simulink model "Modele_LQR_6DOF"  (R2025b)
settings: Solver=VariableStepAuto  StartTime=0.0  StopTime=300  FixedStep=0.033333  RelTol=1e-3
values from neighbouring files (symbols this model uses):
  B = -234.459    [AUV_Params.sldd]    (also in block_compute_K.m = [ [                                          0,             )
  Fx1 = -14.142    [AUV_Params.sldd]
  Fx2 = -14.142    [AUV_Params.sldd]
  Fx3 = 0.0    [AUV_Params.sldd]
  Fx4 = 0.0    [AUV_Params.sldd]
  Fx5 = 0.0    [AUV_Params.sldd]
  Fx6 = 0.0    [AUV_Params.sldd]
  Fx7 = 14.142    [AUV_Params.sldd]
  Fx8 = 14.142    [AUV_Params.sldd]
  Fy1 = 14.142    [AUV_Params.sldd]
  Fy2 = -14.142    [AUV_Params.sldd]
  Fy3 = 0.0    [AUV_Params.sldd]
  Fy4 = 0.0    [AUV_Params.sldd]
  Fy5 = 0.0    [AUV_Params.sldd]
  Fy6 = 0.0    [AUV_Params.sldd]
  Fy7 = 14.142    [AUV_Params.sldd]
  Fy8 = -14.142    [AUV_Params.sldd]
  Fz1 = 0.0    [AUV_Params.sldd]
  Fz2 = 0.0    [AUV_Params.sldd]
  Fz3 = -20.0    [AUV_Params.sldd]
  Fz4 = -20.0    [AUV_Params.sldd]
  Fz5 = -20.0    [AUV_Params.sldd]
  Fz6 = -20.0    [AUV_Params.sldd]
  Fz7 = 0.0    [AUV_Params.sldd]
  Fz8 = 0.0    [AUV_Params.sldd]
  I_x = 0.578    [AUV_Params.sldd]
  I_y = 0.645    [AUV_Params.sldd]
  I_z = 0.9366    [AUV_Params.sldd]
  lx1 = 0.0194    [AUV_Params.sldd]
  lx2 = 0.0194    [AUV_Params.sldd]
  lx3 = -0.0317    [AUV_Params.sldd]
  lx4 = -0.0317    [AUV_Params.sldd]
  lx5 = 0.0317    [AUV_Params.sldd]
  lx6 = 0.0317    [AUV_Params.sldd]
  lx7 = -0.0194    [AUV_Params.sldd]
  lx8 = -0.0194    [AUV_Params.sldd]
  ly1 = 0.0381    [AUV_Params.sldd]
  ly2 = -0.0381    [AUV_Params.sldd]
  ly3 = 0.0049    [AUV_Params.sldd]
  ly4 = -0.0049    [AUV_Params.sldd]
  ly5 = 0.0049    [AUV_Params.sldd]
  ly6 = -0.0049    [AUV_Params.sldd]
  ly7 = 0.0381    [AUV_Params.sldd]
  ly8 = -0.0381    [AUV_Params.sldd]
  lz1 = 0.0575    [AUV_Params.sldd]
  lz2 = 0.0575    [AUV_Params.sldd]
  lz3 = 0.0366    [AUV_Params.sldd]
  lz4 = 0.0366    [AUV_Params.sldd]
  lz5 = 0.0366    [AUV_Params.sldd]
  lz6 = 0.0366    [AUV_Params.sldd]
  lz7 = 0.0575    [AUV_Params.sldd]
  lz8 = 0.0575    [AUV_Params.sldd]
  m = 23.9    [AUV_Params.sldd]
  W = 234.459    [AUV_Params.sldd]
  x_rb = 0.0    [AUV_Params.sldd]
  x_rg = 0.0    [AUV_Params.sldd]
  y_rb = 0.0    [AUV_Params.sldd]
  y_rg = 0.0    [AUV_Params.sldd]
  z_rb = 0.0    [AUV_Params.sldd]
  z_rg = 0.0    [AUV_Params.sldd]
undefined symbols (not defined in the file or in its folder): A_num, Q_envoyer, sigbuilder_block, SIZE_TRAJ, T_TRAJ, TRAJECTOIRE, YAW_MODE
libraries: simulink x12, sharedtransform x1, dspinverses x1, SignalEditorBlockLib x1
(part 3 of 4)

== matlab function Modele_LQR_6DOF/Controller/MATLAB Function ==
  settings: updateMethod=DISCRETE
  data: R output; Q output; A output; B output; state input; Q_files input; A_lineraire input

function [R,Q,A,B]= ABmatrix(state, Q_files, A_lineraire)
tic
    
    roll_ = state(4);
    pitch_ = state(5);
    yaw_ = state(6);
    u = state(7); %
    v = state(8); %
    w = state(9); %
    p = state(10);
    q = state(11);
    r = state(12);
    thrust = 10;
    importance = 0;

    % Q = Q_files;
    Q = diag([Q_files(1,1) Q_files(2,2) Q_files(3,3) Q_files(4,4) Q_files(5,5) Q_files(6,6) Q_files(7,7) Q_files(8,8) Q_files(9,9) Q_files(10,10) Q_files(11,11) Q_files(12,12)]);
    % Q = diag([80, 80, 80, 40, 40, 40, 20, 20, 20, 20, 20, 20]); % test répétition
    % Q = diag([4, 4, 4, 2, 2, 2, 1, 1, 1, 1, 1, 1]); % test ancien
    % R = diag([thrust, thrust, thrust-importance, thrust-importance, thrust-importance, thrust-importance, thrust, thrust]); 
    R = thrust*eye(8);

    radius = 0.26;
    
 % A = A_lineraire;

 A = [[0, 0, 0,   v*(sin(roll_)*sin(yaw_) + cos(roll_)*cos(yaw_)*sin(pitch_)) + w*(cos(roll_)*sin(yaw_) - cos(yaw_)*sin(pitch_)*sin(roll_)), w*cos(pitch_)*cos(roll_)*cos(yaw_) - u*cos(yaw_)*sin(pitch_) + v*cos(pitch_)*cos(yaw_)*sin(roll_), w*(cos(yaw_)*sin(roll_) - cos(roll_)*sin(pitch_)*sin(yaw_)) - v*(cos(roll_)*cos(yaw_) + sin(pitch_)*sin(roll_)*sin(yaw_)) - u*cos(pitch_)*sin(yaw_), cos(pitch_)*cos(yaw_), cos(yaw_)*sin(pitch_)*sin(roll_) - cos(roll_)*sin(yaw_), sin(roll_)*sin(yaw_) + cos(roll_)*cos(yaw_)*sin(pitch_),             0,                      0,                      0]
[0, 0, 0, - v*(cos(yaw_)*sin(roll_) - cos(roll_)*sin(pitch_)*sin(yaw_)) - w*(cos(roll_)*cos(yaw_) + sin(pitch_)*sin(roll_)*sin(yaw_)), w*cos(pitch_)*cos(roll_)*sin(yaw_) - u*sin(pitch_)*sin(yaw_) + v*cos(pitch_)*sin(roll_)*sin(yaw_), w*(sin(roll_)*sin(yaw_) + cos(roll_)*cos(yaw_)*sin(pitch_)) - v*(cos(roll_)*sin(yaw_) - cos(yaw_)*sin(pitch_)*sin(roll_)) + u*cos(pitch_)*cos(yaw_), cos(pitch_)*sin(yaw_), cos(roll_)*cos(yaw_) + sin(pitch_)*sin(roll_)*sin(yaw_), cos(roll_)*sin(pitch_)*sin(yaw_) - cos(yaw_)*sin(roll_),             0,                      0,                      0]
[0, 0, 0,                                                                         v*cos(pitch_)*cos(roll_) - w*cos(pitch_)*sin(roll_),                             - u*cos(pitch_) - w*cos(roll_)*sin(pitch_) - v*sin(pitch_)*sin(roll_),                                                                                                                                                   0,          -sin(pitch_),                                  cos(pitch_)*sin(roll_),                                  cos(pitch_)*cos(roll_),             0,                      0,                      0]
[0, 0, 0,                                                                         q*cos(roll_)*tan(pitch_) - r*tan(pitch_)*sin(roll_),                               r*cos(roll_)*(tan(pitch_)^2 + 1) + q*sin(roll_)*(tan(pitch_)^2 + 1),                                                                                                                                                   0,                     0,                                                       0,                                                       0,             1, tan(pitch_)*sin(roll_), cos(roll_)*tan(pitch_)]
[0, 0, 0,                                                                                               - r*cos(roll_) - q*sin(roll_),                                                                                                 0,                                                                                                                                                   0,                     0,                                                       0,                                                       0,             0,             cos(roll_),            -sin(roll_)]
[0, 0, 0,                                                                     (q*cos(roll_))/cos(pitch_) - (r*sin(roll_))/cos(pitch_),               (r*cos(roll_)*sin(pitch_))/cos(pitch_)^2 + (q*sin(pitch_)*sin(roll_))/cos(pitch_)^2,                                                                                                                                                   0,                     0,                                                       0,                                                       0,             0, sin(roll_)/cos(pitch_), cos(roll_)/cos(pitch_)]
[0, 0, 0,                                                                                                                           0,                                            (10*cos(pitch_)*(13080*pi*radius^3 - 234459/1000))/139,                                                                                                                                                   0,            -2221/1390,                                                       r,                                                      -q,             0,                     -w,                      v]
[0, 0, 0,                                                          -(10*cos(pitch_)*cos(roll_)*(13080*pi*radius^3 - 234459/1000))/139,                                 (10*sin(pitch_)*sin(roll_)*(13080*pi*radius^3 - 234459/1000))/139,                                                                                                                                                   0,                    -r,                                               -1394/695,                                                       p,             w,                      0,                     -u]
[0, 0, 0,                                                           (10*cos(pitch_)*sin(roll_)*(13080*pi*radius^3 - 234459/1000))/139,                                 (10*cos(roll_)*sin(pitch_)*(13080*pi*radius^3 - 234459/1000))/139,                                                                                                                                                   0,                     q,                                                      -p,                                               -2107/695,            -v,                      u,                      0]
[0, 0, 0,                                                                                                                           0,                                                                                                 0,                                                                                                                                                   0,                     0,                                                       0,                                                       0, -193590/40171,           -(146*r)/289,           -(146*q)/289]
[0, 0, 0,                                                                                                                           0,                                                                                                 0,                                                                                                                                                   0,                     0,                                                       0,                                                       0,   (359*r)/645,            -25812/5977,            (359*p)/645]
[0, 0, 0,                                                                                                                           0,                                                                                                 0,                                                                                                                                                   0,                     0,                                                       0,                                                       0,   -(67*q)/937,            -(67*p)/937,         -387180/130243]];

% original
%     A = [[ 0, 0, 0,   v*(sin(roll_)*sin(yaw_) + cos(roll_)*cos(yaw_)*sin(pitch_)) + w*(cos(roll_)*sin(yaw_) - cos(yaw_)*sin(pitch_)*sin(roll_)), w*cos(pitch_)*cos(roll_)*cos(yaw_) - u*cos(yaw_)*sin(pitch_) + v*cos(pitch_)*cos(yaw_)*sin(roll_), w*(cos(yaw_)*sin(roll_) - cos(roll_)*sin(pitch_)*sin(yaw_)) - v*(cos(roll_)*cos(yaw_) + sin(pitch_)*sin(roll_)*sin(yaw_)) - u*cos(pitch_)*sin(yaw_), cos(pitch_)*cos(yaw_), cos(yaw_)*sin(pitch_)*sin(roll_) - cos(roll_)*sin(yaw_), sin(roll_)*sin(yaw_) + cos(roll_)*cos(yaw_)*sin(pitch_),          0,                      0,                      0]
% [ 0, 0, 0, - v*(cos(yaw_)*sin(roll_) - cos(roll_)*sin(pitch_)*sin(yaw_)) - w*(cos(roll_)*cos(yaw_) + sin(pitch_)*sin(roll_)*sin(yaw_)), w*cos(pitch_)*cos(roll_)*sin(yaw_) - u*sin(pitch_)*sin(yaw_) + v*cos(pitch_)*sin(roll_)*sin(yaw_), w*(sin(roll_)*sin(yaw_) + cos(roll_)*cos(yaw_)*sin(pitch_)) - v*(cos(roll_)*sin(yaw_) - cos(yaw_)*sin(pitch_)*sin(roll_)) + u*cos(pitch_)*cos(yaw_), cos(pitch_)*sin(yaw_), cos(roll_)*cos(yaw_) + sin(pitch_)*sin(roll_)*sin(yaw_), cos(roll_)*sin(pitch_)*sin(yaw_) - cos(yaw_)*sin(roll_),          0,                      0,                      0]
% [ 0, 0, 0,                                                                         v*cos(pitch_)*cos(roll_) - w*cos(pitch_)*sin(roll_),                             - u*cos(pitch_) - w*cos(roll_)*sin(pitch_) - v*sin(pitch_)*sin(roll_),                                                                                                                                                   0,          -sin(pitch_),                                  cos(pitch_)*sin(roll_),                                  cos(pitch_)*cos(roll_),          0,                      0,                      0]
% [ 0, 0, 0,                                                                         q*cos(roll_)*tan(pitch_) - r*tan(pitch_)*sin(roll_),                               r*cos(roll_)*(tan(pitch_)^2 + 1) + q*sin(roll_)*(tan(pitch_)^2 + 1),                                                                                                                                                   0,                     0,                                                       0,                                                       0,          1, tan(pitch_)*sin(roll_), cos(roll_)*tan(pitch_)]
% [ 0, 0, 0,                                                                                               - r*cos(roll_) - q*sin(roll_),                                                                                                 0,                                                                                                                                                   0,                     0,                                                       0,                                                       0,          0,             cos(roll_),            -sin(roll_)]
% [ 0, 0, 0,                                                                     (q*cos(roll_))/cos(pitch_) - (r*sin(roll_))/cos(pitch_),               (r*cos(roll_)*sin(pitch_))/cos(pitch_)^2 + (q*sin(pitch_)*sin(roll_))/cos(pitch_)^2,                                                                                                                                                   0,                     0,                                                       0,                                                       0,          0, sin(roll_)/cos(pitch_), cos(roll_)/cos(pitch_)]
% [ 0, 0, 0,                                                                                                                           0,                                                    (7873445366256113*cos(pitch_))/395824185999360,                                                                                                                                                   0,             2221/2250,                                               (17*r)/25,                                          -(1343*q)/2250,          0,         -(1343*w)/2250,              (17*v)/25]
% [ 0, 0, 0,                                                                   -(2315719225369445*cos(pitch_)*cos(roll_))/79164837199872,                                          (2315719225369445*sin(pitch_)*sin(roll_))/79164837199872,                                                                                                                                                   0,            -(25*r)/17,                                                   82/45,                                               (79*p)/90,  (79*w)/90,                      0,             -(25*u)/17]
% [ 0, 0, 0,                                                                      (146564507934775*cos(pitch_)*sin(roll_))/4398046511104,                                            (146564507934775*cos(roll_)*sin(pitch_))/4398046511104,                                                                                                                                                   0,         (2250*q)/1343,                                              -(90*p)/79,                                               4214/1343, -(90*v)/79,          (2250*u)/1343,                      0]
% [ 0, 0, 0,                                                                                                                           0,                                                                                                 0,                                                                                                                                                   0,                     0,                                               (187*w)/4,                                               (187*v)/4,       81/2,                      0,                      0]
% [ 0, 0, 0,                                                                                                                           0,                                                                                                 0,                                                                                                                                                   0,            -(907*w)/4,                                                       0,                                              -(907*u)/4,          0,                   81/2,                      0]
% [ 0, 0, 0,                                                                                                                           0,                                                                                                 0,                                                                                                                                                   0,                 180*v,                                                   180*u,                                                       0,          0,                      0,                   81/2]];


    B = [[                                          0,                                            0,              0,              0,             0,             0,                                            0,                                           0]
[                                          0,                                            0,              0,              0,             0,             0,                                            0,                                           0]
[                                          0,                                            0,              0,              0,             0,             0,                                            0,                                           0]
[                                          0,                                            0,              0,              0,             0,             0,                                            0,                                           0]
[                                          0,                                            0,              0,              0,             0,             0,                                            0,                                           0]
[                                          0,                                            0,              0,              0,             0,             0,                                            0,                                           0]
[                                  -707/6950,                                    -707/6950,              0,              0,             0,             0,                                     707/6950,                                    707/6950]
[                                   707/6950,                                    -707/6950,              0,              0,             0,             0,                                     707/6950,                                   -707/6950]
[                                          0,                                            0,        -20/139,        -20/139,       -20/139,       -20/139,                                            0,                                           0]
[                                          0,                                            0,  -130255/80342,   130255/80342, -130255/80342,  130255/80342,                                            0,                                           0]
[                                          0,                                            0, -256447/448275, -256447/448275, 256447/448275, 256447/448275,                                            0,                                           0]
[194698457386957391875/146640581566903877632, -194698457386957391875/146640581566903877632,              0,              0,             0,             0, -194698457386957391875/146640581566903877632, 194698457386957391875/146640581566903877632]];

% matrice original
%     B = [[                                   0,                                    0,         0,         0,         0,         0,                                    0,                                   0]
% [                                   0,                                    0,         0,         0,         0,         0,                                    0,                                   0]
% [                                   0,                                    0,         0,         0,         0,         0,                                    0,                                   0]
% [                                   0,                                    0,         0,         0,         0,         0,                                    0,                                   0]
% [                                   0,                                    0,         0,         0,         0,         0,                                    0,                                   0]
% [                                   0,                                    0,         0,         0,         0,         0,                                    0,                                   0]
% [                          -707/11250,                           -707/11250,         0,         0,         0,         0,                            707/11250,                           707/11250]
% [                            707/7650,                            -707/7650,         0,         0,         0,         0,                             707/7650,                           -707/7650]
% [                                   0,                                    0, -200/1343, -200/1343, -200/1343, -200/1343,                                    0,                                   0]
% [                                   0,                                    0,    -109/8,     109/8,    -109/8,     109/8,                                    0,                                   0]
% [                                   0,                                    0, -1073/200, -1073/200,  1073/200,  1073/200,                                    0,                                   0]
% [ 162927579403311625/9007199254740992, -162927579403311625/9007199254740992,         0,         0,         0,         0, -162927579403311625/9007199254740992, 162927579403311625/9007199254740992]];

toc
end

== matlab function Modele_LQR_6DOF/Thrustherforces in newtons/MATLAB Function1 ==
  data: u input; y output
function y = Normalize(u)
y = (u-1500)*150/400;

== matlab function Modele_LQR_6DOF/ROV model/ROV model/Kinematics ==
  data: u_b input; u_n output; v_b input; w_b input; p_b input; q_b input; r_b input; phi input; theta input; psi input; v_n output; w_n output; p_n output; q_n output; r_n output
function [u_n,v_n,w_n,p_n,q_n,r_n] = Kinematics(u_b,v_b,w_b,p_b,q_b,r_b,phi,theta,psi)
% LIVRE HMCH PAGE 27
cphi = cos(phi);
sphi = sin(phi);
cth  = cos(theta);
sth  = sin(theta);
cpsi = cos(psi);
spsi = sin(psi);
tanth = tan(theta);
if cth==0
    error('T is singular for theta = +-90 degrees');
end
 
u_n = u_b*cpsi*cth + v_b*(cpsi*sphi*sth - cphi*spsi) + w_b*(sphi*spsi + cphi*cpsi*sth) ;
v_n = u_b*cth*spsi + v_b*(cphi*cpsi + sphi*spsi*sth) + w_b*(cphi*spsi*sth - cpsi*sphi);
w_n = -u_b*sth+ v_b*cth*sphi + w_b*cphi*cth;
p_n = p_b + q_b*sphi*(tanth) + r_b*cphi*(tanth);
q_n = q_b*cphi - r_b*sphi;
r_n = q_b*(sphi/cth) + r_b*(cphi/cth);

% u_n =  w_b*(sphi*spsi + cphi*cpsi*sth) - v_b*(cphi*spsi - cpsi*sphi*sth) + u_b*cpsi*cth;
% v_n =  v_b*(cphi*cpsi + sphi*spsi*sth) - w_b*(cpsi*sphi - cphi*spsi*sth) + u_b*cth*spsi;
% w_n = w_b*cphi*cth - u_b*sth + v_b*cth*sphi;
% p_n = p_b + (r_b*cphi*sth)/cth + (q_b*sphi*sth)/cth;
% q_n = q_b*cphi - r_b*sphi;
% r_n = (r_b*cphi)/cth + (q_b*sphi)/cth;
end

== matlab function Modele_LQR_6DOF/Controller/LQR/MATLAB Function ==
  settings: updateMethod=DISCRETE
  data: dXdt output; X input; A input; B input; R input; Q input
function dXdt  = mRiccati(X, A, B,R,Q)
% r1=randi([1 1000]);
% r2=randi([1 1000]);
% r3=randi([1 1000]);
% r4=randi([1 1000]);
% r5=randi([1 1000]);
% r6=randi([1 1000]);
% Q = diag([r1 r2 r3 r4 r5 r6] );
% R = 1*diag([1 1 1 1]);
%X = reshape(X, size(A)); %Convert from "n^2"-by-1 to "n"-by-"n"
dXdt = A.'*X + X*A - (X*B)*inv(R)*(B.'*X) + Q; %Determine derivative
% dXdtS= dXdt(:); %Convert from "n"-by-"n" to "n^2"-by-1,algebraic Riccati equation (ARE)

== matlab function Modele_LQR_6DOF/MATLAB Function ==
  data: Position input; srf_in input
function Visualize(Position, srf_in)

    coder.extrinsic('setax'); 
    setax(Position, srf_in);  

end

== matlab function Modele_LQR_6DOF/Controller/Gestionnaire des Vitesses/MATLAB Function2 ==
  data: xstate input; u output; xtarget input
function u = fcn(xstate,xtarget)

precition = 0.01;
% precition = 0.01; % original

if(xstate < xtarget - precition)
    u = 1; % original (1)

elseif(xstate > xtarget + precition)
    u = -1; % original (-1)
    
else
    u = 0;
end
end

== matlab function Modele_LQR_6DOF/Controller/Gestionnaire des Vitesses/MATLAB Function3 ==
  data: xstate input; u output; xtarget input
function u = fcn(xstate,xtarget)

precition = 0.05;
% precition = 0.05; % original

if(xstate < xtarget - precition)
    u = 0.5; % 0.5

elseif(xstate > xtarget + precition)
    u = -0.5;
    
else
    u = 0;
end
end

== matlab function Modele_LQR_6DOF/Controller/Gestionnaire des Vitesses/MATLAB Function4 ==
  data: xstate input; u output; xtarget input
function u = fcn(xstate,xtarget)

precition = 0.05;
% precition = 0.05; % original

if(xstate < xtarget - precition)
    u = 0.5; % 0.5

elseif(xstate > xtarget + precition)
    u = -0.5;
    
else
    u = 0;
end
end

== matlab function Modele_LQR_6DOF/Controller/Gestionnaire des Vitesses/MATLAB Function5 ==
  data: xstate input; u output; xtarget input
function u = fcn(xstate,xtarget)

precition = 0.02;
% precition = 0.02; % originalt

if(xstate < xtarget - precition)
    u = 0.2; % avant 0.2

elseif(xstate > xtarget + precition)
    u = -0.2;
    
else
    u = 0;
end
end

== matlab function Modele_LQR_6DOF/Subsystem/MATLAB Function ==
  data: y input; angle output; x input; position input
function angle  = fcn(y, x, position)

persistent x_sub y_sub

% Initialiser la position actuelle si première exécution
if isempty(x_sub)
    x_sub = 0;
    y_sub = 0;
end
angle = 0;

if position(1) >= 1 && position(2) <= 1
    angle = pi/2;
end
if position(1) >= 1 && position(2) >= 1
    angle = pi;
end
if position(1) <= 1 && position(2) >= 1
    angle = pi/2;
end
if position(1) <= 1 && position(2) <= 1
    angle = 0;
end




% % Calculer le vecteur vers la commande
% dx = x - position(1);
% dy = y - position(2);
% 
% % Calculer l'angle avec atan2
% 
% angle = atan2(dy, dx);


% Normaliser entre 0 et 2*pi
% angle = mod(angle, 2*pi);




end

== matlab function Modele_LQR_6DOF/Subsystem/MATLAB Function1 ==
  data: t input; x_ref output; y_ref output; TRAJECTOIRE input; yaw_ref output; YAW_MODE input; T_TRAJ input; SIZE_TRAJ input
function [x_ref, y_ref, yaw_ref] = trajectoire(t, TRAJECTOIRE, YAW_MODE, T_TRAJ, SIZE_TRAJ)
switch int32(TRAJECTOIRE)
    case 1  % carre — cote = SIZE_TRAJ
        T       = T_TRAJ;
        a       = SIZE_TRAJ;
        px      = T * (1.5/30);
        py      = T * (8.5/30);
        x_ref   = onde_carree(t, a, T, 0.50, px);
        y_ref   = onde_carree(t, a, T, 0.50, py);
        yaw_raw = yaw_carre(t, T, 0.50, px, py);

    case 2  % cercle — rayon = SIZE_TRAJ
        R       = SIZE_TRAJ;
        omega   = 2*pi / T_TRAJ;
        x_ref   = R * sin(omega * t);
        y_ref   = R * (1 - cos(omega * t));
        yaw_raw = atan2(sin(omega*t), cos(omega*t));

    case 3  % Lissajous — amplitude = SIZE_TRAJ
        A       = SIZE_TRAJ;
        omega1  = 2 * (2*pi / T_TRAJ);
        omega2  = omega1 * 1.61803;
        x_ref   = A * sin(omega1*t) * cos(omega2*t);
        y_ref   = A * sin(omega1*t) * sin(omega2*t);
        dx      = A*(omega1*cos(omega1*t)*cos(omega2*t) - omega2*sin(omega1*t)*sin(omega2*t));
        dy      = A*(omega1*cos(omega1*t)*sin(omega2*t) + omega2*sin(omega1*t)*cos(omega2*t));
        yaw_raw = atan2(dy, dx);

    otherwise
        x_ref = 0.0;  y_ref = 0.0;  yaw_raw = 0.0;
end

yaw_ref = double(int32(YAW_MODE)) * yaw_raw;
end

function yaw = yaw_carre(t, T, duty, px, py)
t_y1r = py - px;
t_x0r = duty * T;
t_y0r = (py - px) + duty * T;
if t < px
    yaw = 0.0;
else
    tn = mod(t - px, T);
    if     tn < t_y1r,  yaw = 0.0;
    elseif tn < t_x0r,  yaw = pi/2;
    elseif tn < t_y0r,  yaw = pi;
    else,               yaw = -pi/2;
    end
end
end

function y = onde_carree(t, amplitude, periode, duty, phase)
t_adj = t - phase;
if t_adj <= 0,  y = 0.0;
else,  y = amplitude * double(mod(t_adj, periode) < duty * periode);
end
end

== matlab function Modele_LQR_6DOF/Controller/MATLAB Function2 ==
  data: K input; u output; state input; target_state input
function u = State_error(K,state,target_state)
u = zeros(8,1);
u = -K*(state-target_state);
end
